simulink model "hw2_p8_b"  (R2020a)
settings: Solver=VariableStepAuto  StartTime=0.0  StopTime=10  RelTol=1e-3
settings Model: Creator=Tomo  LastModifiedBy=Tomo

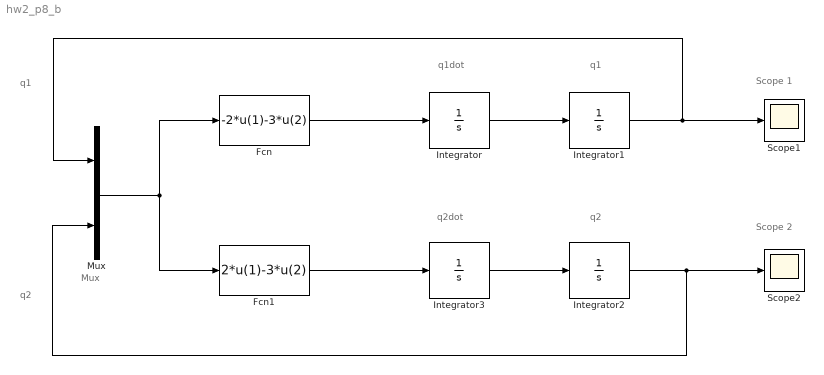
== system hw2_p8_b ==
  note: q1dot
  note: Mux
  note: q2
  note: q2
  note: q2dot
  note: q1
  note: Scope 1
  note: q1
  note: Scope 2
  Fcn : Fcn  Expr=-2*u(1)-3*u(2)
  Fcn1 : Fcn  Expr=2*u(1)-3*u(2)
  Integrator : Integrator
  Integrator1 : Integrator  InitialCondition=0.8
  Integrator2 : Integrator  InitialCondition=0.2
  Integrator3 : Integrator
  Mux : Mux  Inputs=2
  Scope1 : Scope
  Scope2 : Scope
  wires:
  Mux/1 -> Fcn1/1, Fcn/1
  Integrator/1 -> Integrator1/1
  Integrator3/1 -> Integrator2/1
  Fcn/1 -> Integrator/1
  Integrator1/1 -> Mux/1, Scope1/1
  Integrator2/1 -> Mux/2, Scope2/1
  Fcn1/1 -> Integrator3/1
